simulink model "chydrbf_bruite_z_ss"  (R2025b)
settings: Solver=ode45  StartTime=0.0  StopTime=50  MaxStep=1  MinStep=0.0001  RelTol=1e-8  AbsTol=1e-8  EnableMultiTasking=on
values from neighbouring files (symbols this model uses):
  Aobs = aad-Ld*cad    [initchydr_yuwch.m]
  Bobs = [bad Ld]    [initchydr_yuwch.m]
  Cobs = eye(5)    [initchydr_yuwch.m]
  Dobs = zeros(5,2)    [initchydr_yuwch.m]
  Kd = place(ad,bd_u, roots(Cd))    [initchydr_yuwch.m]
  Kdc = inv(cd*inv(eye(4)-ad+bd_u*Kd)*bd_u)    [initchydr_yuwch.m]
  Kdp = -inv(cd*inv(eye(4)-ad+bd_u*Kd)*bd_u)*cd*inv(eye(4)-ad+bd_u*Kd)*bd_p    [initchydr_yuwch.m]
  kw = 0.5    [datahydr_pprTf5.mat]    (also in initchydr_yuwch.m)
  Ta = 10    [datahydr_pprTf5.mat]    (also in initchydr_yuwch.m)
  Te = 0.4    [initchydr_yuwch.m]
  TI = 0.3    [datahydr_pprTf5.mat]    (also in initchydr_yuwch.m)
  Tw = 1    [datahydr_pprTf5.mat]    (also in initchydr_yuwch.m)
settings Model: Creator=pchevrel  LastModifiedBy=flo
settings SolverCC: AutoScaleAbsTol=off  AlgebraicLoopSolver=TrustRegion
settings DataIOCC: LimitDataPoints=on  SaveFormat=Array  SignalLoggingSaveFormat=ModelDataLogs  SaveOutput=off  SaveTime=off  ReturnWorkspaceOutputs=off  SignalLoggingName=sigsOut
settings OptimizationCC: ExpressionDepthLimit=2147483647.0  InitFltsAndDblsToZero=on  LifeSpan=inf
settings DebuggingCC: SaveWithParameterizedLinksMsg=none  UnderspecifiedInitializationDetection=Classic  MergeDetectMultiDrivingBlocksExec=none  SignalResolutionControl=TryResolveAllWithWarning  MultiTaskDSMMsg=warning  MultiTaskCondExecSysMsg=none  FcnCallInpInsideContextMsg=warning  UnconnectedInputMsg=warning  UnconnectedOutputMsg=warning  UnconnectedLineMsg=warning  StateNameClashWarn=warning  SFUnexpectedBacktrackingDiag=warning  SFNoUnconditionalDefaultTransitionDiag=warning  SFExecutionAtInitializationDiag=none  ArithmeticOperatorsInVariantConditions=warning
settings HardwareCC: ProdBitPerPointer=32.0  ProdBitPerSizeT=32.0  ProdBitPerPtrDiffT=32.0  ProdLargestAtomicFloat=None  ProdIntDivRoundTo=Undefined  ProdEndianess=Unspecified  ProdWordSize=32.0  ProdHWDeviceType=32-bit Generic  TargetUnknown=on
settings ModelReferenceCC: EnableRefExpFcnMdlSchedulingChecks=on  PropagateSignalLabelsOutOfModel=off
settings SFSimCC: SimUseLocalCustomCode=off  CustomCodeUndefinedFunction=UseInterfaceOnly
settings RTWCC: RTWUseLocalCustomCode=off  GPUComputeCapability=3.5  DLArmComputeVersion=19.05
settings CodeAppCC: StateflowObjectComments=on
settings GRTTargetCC: TargetFcnLib=ansi_tfl_tmw.mat  TargetLangStandard=C89/C90 (ANSI)  CombineOutputUpdateFcns=off  GRTInterface=on
settings ConfigComp: CovMetricSettings=dw  CovSaveCumulativeToWorkspaceVar=on  CovSaveSingleToWorkspaceVar=on  CovExternalEMLEnable=off

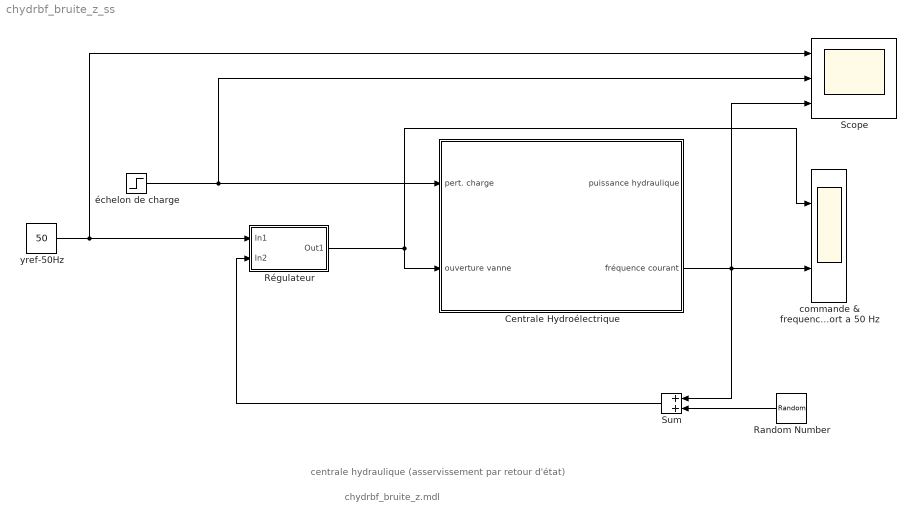
== system chydrbf_bruite_z_ss ==
  note: chydrbf_bruite_z.mdl
  note: centrale hydraulique (asservissement par retour d'état)
  Centrale Hydroélectrique : Subsystem
  Random Number : RandomNumber  Variance=5  SampleTime=0
  Régulateur : Subsystem
  Scope : Scope  NumInputPorts=3
      settings: ActiveDisplayYMinimum=-7.0299882777816673  ActiveDisplayYMaximum=57.682578630725359
  Sum : Sum  InputSameDT=on  SaturateOnIntegerOverflow=on  OutDataTypeStr=Inherit: Same as first input
  commande & frequence en relatif par rapport a 50 Hz : Scope  NumInputPorts=2
      settings: ActiveDisplayYMinimum=-25.468942060309637  ActiveDisplayYMaximum=174.06733877909735
  yref-50Hz : Constant  Value=50
  échelon de charge : Step  Time=20  After=10  SampleTime=0
  wires:
  Centrale Hydroélectrique/2(fréquence courant) -> Scope/3, commande & frequence en relatif par rapport a 50 Hz/2, Sum/1
  yref-50Hz/1 -> Régulateur/1(In1), Scope/1
  échelon de charge/1 -> Scope/2, Centrale Hydroélectrique/1(pert. charge)
  Random Number/1 -> Sum/2
  Régulateur/1(Out1) -> Centrale Hydroélectrique/2(ouverture vanne), commande & frequence en relatif par rapport a 50 Hz/1
  Sum/1 -> Régulateur/2(In2)

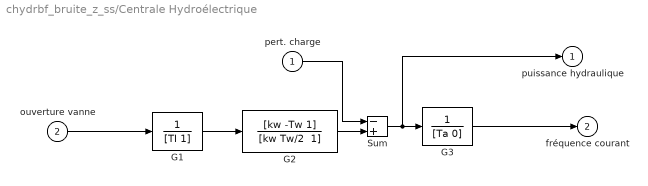
== system chydrbf_bruite_z_ss/Centrale Hydroélectrique ==
  pert. charge : Inport
  ouverture vanne : Inport  Port=2
  G1 : TransferFcn  Denominator=[TI 1]
  G2 : TransferFcn  Numerator=[kw -Tw 1]  Denominator="[kw Tw/2  1]"
  G3 : TransferFcn  Denominator=[Ta 0]
  Sum : Sum  Inputs=-+  InputSameDT=on  SaturateOnIntegerOverflow=on  OutDataTypeStr=Inherit: Same as first input
  puissance hydraulique : Outport
  fréquence courant : Outport  Port=2
  wires:
  G2/1 -> Sum/2
  Sum/1 -> G3/1, puissance hydraulique/1
  G3/1 -> fréquence courant/1
  G1/1 -> G2/1
  pert. charge/1 -> Sum/1
  ouverture vanne/1 -> G1/1

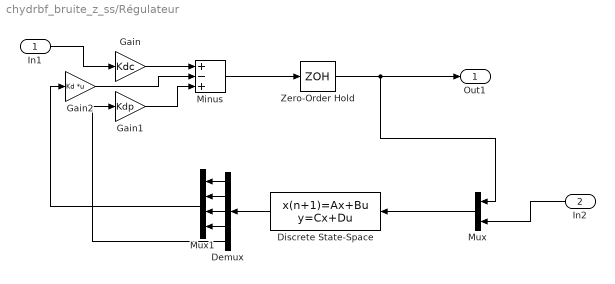
== system chydrbf_bruite_z_ss/Régulateur ==
  In1 : Inport
  In2 : Inport  Port=2
  Demux : Demux  Outputs=5
  Discrete State-Space : DiscreteStateSpace  A=Aobs  B=Bobs  C=Cobs  D=Dobs  SampleTime=Te
  Gain : Gain  Gain=Kdc
  Gain1 : Gain  Gain=Kdp
  Gain2 : Gain  Gain=Kd  Multiplication=Matrix(K*u)
  Minus : Sum  Inputs=+-+
  Mux : Mux  Inputs=2
  Mux1 : Mux
  Zero-Order Hold : ZeroOrderHold  SampleTime=Te
  Out1 : Outport
  wires:
  Minus/1 -> Zero-Order Hold/1
  Demux/1 -> Mux1/1
  Gain/1 -> Minus/1
  In1/1 -> Gain/1
  Mux/1 -> Discrete State-Space/1
  Demux/2 -> Mux1/2
  Demux/3 -> Mux1/3
  Discrete State-Space/1 -> Demux/1
  Demux/4 -> Mux1/4
  Demux/5 -> Gain1/1
  Gain2/1 -> Minus/2
  Mux1/1 -> Gain2/1
  Zero-Order Hold/1 -> Mux/1, Out1/1
  Gain1/1 -> Minus/3
  In2/1 -> Mux/2
